simulink model "directVectorControl"  (R2021a)
settings: Solver=FixedStepAuto  StartTime=0.0  StopTime=10  FixedStep=1e-6  RelTol=1e-3
InitFcn:
  | Rs=1.405;
  | Lls=0.005839;
  | rr=1.395;
  | Llr=0.005839;
  | Lm=0.1722;
  | Lr=Llr+Lm;
  | J=0.0131;
  | B=0.002985;
  | p=4;
  | Tl=2;
  | Lr=Llr+Lm;
  | Taur=Lr/rr;
  | P = p;
  | Ls = Lls + Lm;
  | Lr = Llr + Lm;
  | Rr = rr;
  | w_frame = 2*pi*50;
  | Vdc=650;
  | car_freq=10000;
  | Rotor_Flux=0.9;
  | Delta=0.1;
libraries: pid_lib x14, spsIGBTDiodeLib x6, spsabctodq0Lib x5, eeStairGenerator x3, spsdq0toabcLib x3, spsVoltageMeasurementLib x3, spsGroundLib x2, spsDCVoltageSourceLib x1, spsAsynchronousMachineSIUnitsLib x1, spsTriangleGeneratorLib x1, spspowerguiLib x1
(part 2 of 2)

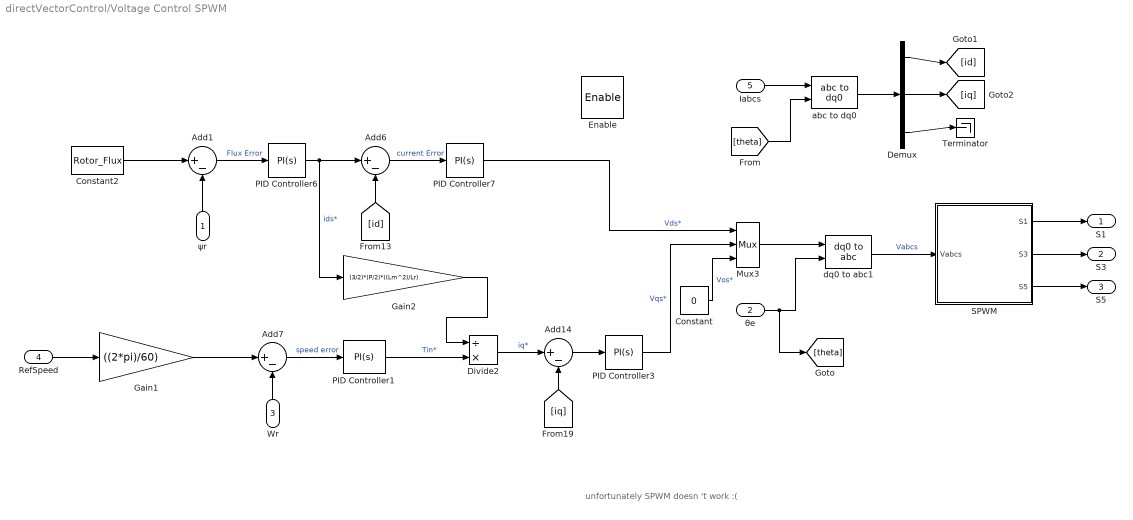
== system directVectorControl/Voltage Control SPWM ==
  note: unfortunately SPWM doesn 't work :(
  ψr : Inport
  θe : Inport  Port=2
  Wr : Inport  Port=3
  RefSpeed : Inport  Port=4
  Iabcs : Inport  Port=5
  Enable : EnablePort
  Add{1,6..7,14} (4 alike) : Sum  Inputs=|+-
  Constant : Constant  Value=0
  Constant2 : Constant  Value=Rotor_Flux
  Demux : Demux  Outputs=3
  Divide2 : Product  Inputs=/*
  Gain1 : Gain  Gain=((2*pi)/60)
  Gain2 : Gain  Gain=(3/2)*(P/2)*((Lm^2)/Lr)
  Mux3 : Mux  Inputs=3
      settings: DisplayOption=signals
  PID Controller1 : pid_lib/PID Controller  Controller=PI  Form=Parallel  TimeDomain=Continuous-time  UseExternalTs=off  SampleTime=-1  IntegratorMethod=Forward Euler  FilterMethod=Forward Euler  ControllerParametersSource=internal  P=107.29735671651  I=38872.1307396283  D=0  UseFilter=on  N=100  TunerSelectOption=Transfer Function Based (PID Tuner App)  InitialConditionSource=internal  InitialConditionForIntegrator=0  InitialConditionForFilter=0  DifferentiatorICPrevScaledInput=0  ExternalReset=none  TrackingMode=off  Kt=1  LimitOutput=off  SatLimitsSource=internal  UpperSaturationLimit=26  LowerSaturationLimit=0  LinearizeAsGain=on  AntiWindupMode=none  Kb=1  POutMin=[]  POutMax=[]  IOutMin=[]  IOutMax=[]  DOutMin=[]  DOutMax=[]  NOutMin=[]  NOutMax=[]  SumOutMin=[]  SumOutMax=[]  SaturationOutMin=[]  SaturationOutMax=[]  PParamMin=[]  PParamMax=[]  IParamMin=[]  IParamMax=[]  DParamMin=[]  DParamMax=[]  NParamMin=[]  NParamMax=[]  KbParamMin=[]  KbParamMax=[]  KtParamMin=[]  KtParamMax=[]  KbOutMin=[]  KbOutMax=[]  KtOutMin=[]  KtOutMax=[]  IntegratorOutMin=[]  IntegratorOutMax=[]  FilterOutMin=[]  FilterOutMax=[]  SumI1OutMin=[]  SumI1OutMax=[]  SumI2OutMin=[]  SumI2OutMax=[]  SumI3OutMin=[]  SumI3OutMax=[]  SumI4OutMin=[]  SumI4OutMax=[]  SumDOutMin=[]  SumDOutMax=[]  DifferentiatorOutMin=[]  DifferentiatorOutMax=[]  FilterDiffOutCoefMin=[]  FilterDiffOutCoefMax=[]  ReciprocalOutMin=[]  ReciprocalOutMax=[]  SumDenOutMin=[]  SumDenOutMax=[]  SumNumOutMin=[]  SumNumOutMax=[]  DivideOutMin=[]  DivideOutMax=[]  UdiffTsProdOutMin=[]  UdiffTsProdOutMax=[]  NTsProdOutMin=[]  NTsProdOutMax=[]  UintegralTsProdOutMin=[]  UintegralTsProdOutMax=[]  UngainTsProdOutMin=[]  UngainTsProdOutMax=[]  IntegratorContinuousStateAttributes=''  IntegratorStateMustResolveToSignalObject=off  IntegratorRTWStateStorageClass=Auto  FilterContinuousStateAttributes=''  FilterStateMustResolveToSignalObject=off  FilterRTWStateStorageClass=Auto  ParallelPVariant=InternalParameters  IdealPVariant=Disabled  IVariant=InternalParameters  DVariant=Disabled  IntegratorVariant=Continuous  SatVariant=Disabled  AWVariant=Passthrough  PCopyVariant=Disabled  TRVariant=Disabled  FdbkBlocksVariant=Forward  IdealPFdbkVariant=Disabled  SatFdbkVariant=Disabled  DerivativeFilterVariant=Disabled  NVariant=Disabled  NCopyVariant=Disabled_SignalSpec  FilterICVariant=Disabled  IntegratorICVariant=InternalICs  ExternalResetVariant=Disabled  TRSumVariant=Passthrough  SumFdbkVariant=Disabled  SumVariant=Sum_PI  TsampFilterVariant=InternalTs  TsampNgainVariant=Passthrough  TsampIntegralVariant=Passthrough  ExternalSaturationOutDataTypeStr=Inherit: Same as second input
  PID Controller3 : pid_lib/PID Controller  Controller=PI  Form=Parallel  TimeDomain=Continuous-time  UseExternalTs=off  SampleTime=-1  IntegratorMethod=Forward Euler  FilterMethod=Forward Euler  ControllerParametersSource=internal  P=417.900587639527  I=299199.169732292  D=0  UseFilter=on  N=100  TunerSelectOption=Transfer Function Based (PID Tuner App)  InitialConditionSource=internal  InitialConditionForIntegrator=0  InitialConditionForFilter=0  DifferentiatorICPrevScaledInput=0  ExternalReset=none  TrackingMode=off  Kt=1  LimitOutput=off  SatLimitsSource=internal  UpperSaturationLimit=inf  LowerSaturationLimit=-inf  LinearizeAsGain=on  AntiWindupMode=none  Kb=1  POutMin=[]  POutMax=[]  IOutMin=[]  IOutMax=[]  DOutMin=[]  DOutMax=[]  NOutMin=[]  NOutMax=[]  SumOutMin=[]  SumOutMax=[]  SaturationOutMin=[]  SaturationOutMax=[]  PParamMin=[]  PParamMax=[]  IParamMin=[]  IParamMax=[]  DParamMin=[]  DParamMax=[]  NParamMin=[]  NParamMax=[]  KbParamMin=[]  KbParamMax=[]  KtParamMin=[]  KtParamMax=[]  KbOutMin=[]  KbOutMax=[]  KtOutMin=[]  KtOutMax=[]  IntegratorOutMin=[]  IntegratorOutMax=[]  FilterOutMin=[]  FilterOutMax=[]  SumI1OutMin=[]  SumI1OutMax=[]  SumI2OutMin=[]  SumI2OutMax=[]  SumI3OutMin=[]  SumI3OutMax=[]  SumI4OutMin=[]  SumI4OutMax=[]  SumDOutMin=[]  SumDOutMax=[]  DifferentiatorOutMin=[]  DifferentiatorOutMax=[]  FilterDiffOutCoefMin=[]  FilterDiffOutCoefMax=[]  ReciprocalOutMin=[]  ReciprocalOutMax=[]  SumDenOutMin=[]  SumDenOutMax=[]  SumNumOutMin=[]  SumNumOutMax=[]  DivideOutMin=[]  DivideOutMax=[]  UdiffTsProdOutMin=[]  UdiffTsProdOutMax=[]  NTsProdOutMin=[]  NTsProdOutMax=[]  UintegralTsProdOutMin=[]  UintegralTsProdOutMax=[]  UngainTsProdOutMin=[]  UngainTsProdOutMax=[]  IntegratorContinuousStateAttributes=''  IntegratorStateMustResolveToSignalObject=off  IntegratorRTWStateStorageClass=Auto  FilterContinuousStateAttributes=''  FilterStateMustResolveToSignalObject=off  FilterRTWStateStorageClass=Auto  ParallelPVariant=InternalParameters  IdealPVariant=Disabled  IVariant=InternalParameters  DVariant=Disabled  IntegratorVariant=Continuous  SatVariant=Disabled  AWVariant=Passthrough  PCopyVariant=Disabled  TRVariant=Disabled  FdbkBlocksVariant=Forward  IdealPFdbkVariant=Disabled  SatFdbkVariant=Disabled  DerivativeFilterVariant=Disabled  NVariant=Disabled  NCopyVariant=Disabled_SignalSpec  FilterICVariant=Disabled  IntegratorICVariant=InternalICs  ExternalResetVariant=Disabled  TRSumVariant=Passthrough  SumFdbkVariant=Disabled  SumVariant=Sum_PI  TsampFilterVariant=InternalTs  TsampNgainVariant=Passthrough  TsampIntegralVariant=Passthrough  ExternalSaturationOutDataTypeStr=Inherit: Same as second input
  PID Controller6 : pid_lib/PID Controller  Controller=PI  Form=Parallel  TimeDomain=Continuous-time  UseExternalTs=off  SampleTime=-1  IntegratorMethod=Forward Euler  FilterMethod=Forward Euler  ControllerParametersSource=internal  P=1630.03954669268  I=566675.517481641  D=0  UseFilter=on  N=100  TunerSelectOption=Transfer Function Based (PID Tuner App)  InitialConditionSource=internal  InitialConditionForIntegrator=0  InitialConditionForFilter=0  DifferentiatorICPrevScaledInput=0  ExternalReset=none  TrackingMode=off  Kt=1  LimitOutput=off  SatLimitsSource=internal  UpperSaturationLimit=inf  LowerSaturationLimit=-inf  LinearizeAsGain=on  AntiWindupMode=none  Kb=1  POutMin=[]  POutMax=[]  IOutMin=[]  IOutMax=[]  DOutMin=[]  DOutMax=[]  NOutMin=[]  NOutMax=[]  SumOutMin=[]  SumOutMax=[]  SaturationOutMin=[]  SaturationOutMax=[]  PParamMin=[]  PParamMax=[]  IParamMin=[]  IParamMax=[]  DParamMin=[]  DParamMax=[]  NParamMin=[]  NParamMax=[]  KbParamMin=[]  KbParamMax=[]  KtParamMin=[]  KtParamMax=[]  KbOutMin=[]  KbOutMax=[]  KtOutMin=[]  KtOutMax=[]  IntegratorOutMin=[]  IntegratorOutMax=[]  FilterOutMin=[]  FilterOutMax=[]  SumI1OutMin=[]  SumI1OutMax=[]  SumI2OutMin=[]  SumI2OutMax=[]  SumI3OutMin=[]  SumI3OutMax=[]  SumI4OutMin=[]  SumI4OutMax=[]  SumDOutMin=[]  SumDOutMax=[]  DifferentiatorOutMin=[]  DifferentiatorOutMax=[]  FilterDiffOutCoefMin=[]  FilterDiffOutCoefMax=[]  ReciprocalOutMin=[]  ReciprocalOutMax=[]  SumDenOutMin=[]  SumDenOutMax=[]  SumNumOutMin=[]  SumNumOutMax=[]  DivideOutMin=[]  DivideOutMax=[]  UdiffTsProdOutMin=[]  UdiffTsProdOutMax=[]  NTsProdOutMin=[]  NTsProdOutMax=[]  UintegralTsProdOutMin=[]  UintegralTsProdOutMax=[]  UngainTsProdOutMin=[]  UngainTsProdOutMax=[]  IntegratorContinuousStateAttributes=''  IntegratorStateMustResolveToSignalObject=off  IntegratorRTWStateStorageClass=Auto  FilterContinuousStateAttributes=''  FilterStateMustResolveToSignalObject=off  FilterRTWStateStorageClass=Auto  ParallelPVariant=InternalParameters  IdealPVariant=Disabled  IVariant=InternalParameters  DVariant=Disabled  IntegratorVariant=Continuous  SatVariant=Disabled  AWVariant=Passthrough  PCopyVariant=Disabled  TRVariant=Disabled  FdbkBlocksVariant=Forward  IdealPFdbkVariant=Disabled  SatFdbkVariant=Disabled  DerivativeFilterVariant=Disabled  NVariant=Disabled  NCopyVariant=Disabled_SignalSpec  FilterICVariant=Disabled  IntegratorICVariant=InternalICs  ExternalResetVariant=Disabled  TRSumVariant=Passthrough  SumFdbkVariant=Disabled  SumVariant=Sum_PI  TsampFilterVariant=InternalTs  TsampNgainVariant=Passthrough  TsampIntegralVariant=Passthrough  ExternalSaturationOutDataTypeStr=Inherit: Same as second input
  PID Controller7 : pid_lib/PID Controller  Controller=PI  Form=Parallel  TimeDomain=Continuous-time  UseExternalTs=off  SampleTime=-1  IntegratorMethod=Forward Euler  FilterMethod=Forward Euler  ControllerParametersSource=internal  P=15.9312047333312  I=78964.3934467361  D=0  UseFilter=on  N=100  TunerSelectOption=Transfer Function Based (PID Tuner App)  InitialConditionSource=internal  InitialConditionForIntegrator=0  InitialConditionForFilter=0  DifferentiatorICPrevScaledInput=0  ExternalReset=none  TrackingMode=off  Kt=1  LimitOutput=off  SatLimitsSource=internal  UpperSaturationLimit=inf  LowerSaturationLimit=-inf  LinearizeAsGain=on  AntiWindupMode=none  Kb=1  POutMin=[]  POutMax=[]  IOutMin=[]  IOutMax=[]  DOutMin=[]  DOutMax=[]  NOutMin=[]  NOutMax=[]  SumOutMin=[]  SumOutMax=[]  SaturationOutMin=[]  SaturationOutMax=[]  PParamMin=[]  PParamMax=[]  IParamMin=[]  IParamMax=[]  DParamMin=[]  DParamMax=[]  NParamMin=[]  NParamMax=[]  KbParamMin=[]  KbParamMax=[]  KtParamMin=[]  KtParamMax=[]  KbOutMin=[]  KbOutMax=[]  KtOutMin=[]  KtOutMax=[]  IntegratorOutMin=[]  IntegratorOutMax=[]  FilterOutMin=[]  FilterOutMax=[]  SumI1OutMin=[]  SumI1OutMax=[]  SumI2OutMin=[]  SumI2OutMax=[]  SumI3OutMin=[]  SumI3OutMax=[]  SumI4OutMin=[]  SumI4OutMax=[]  SumDOutMin=[]  SumDOutMax=[]  DifferentiatorOutMin=[]  DifferentiatorOutMax=[]  FilterDiffOutCoefMin=[]  FilterDiffOutCoefMax=[]  ReciprocalOutMin=[]  ReciprocalOutMax=[]  SumDenOutMin=[]  SumDenOutMax=[]  SumNumOutMin=[]  SumNumOutMax=[]  DivideOutMin=[]  DivideOutMax=[]  UdiffTsProdOutMin=[]  UdiffTsProdOutMax=[]  NTsProdOutMin=[]  NTsProdOutMax=[]  UintegralTsProdOutMin=[]  UintegralTsProdOutMax=[]  UngainTsProdOutMin=[]  UngainTsProdOutMax=[]  IntegratorContinuousStateAttributes=''  IntegratorStateMustResolveToSignalObject=off  IntegratorRTWStateStorageClass=Auto  FilterContinuousStateAttributes=''  FilterStateMustResolveToSignalObject=off  FilterRTWStateStorageClass=Auto  ParallelPVariant=InternalParameters  IdealPVariant=Disabled  IVariant=InternalParameters  DVariant=Disabled  IntegratorVariant=Continuous  SatVariant=Disabled  AWVariant=Passthrough  PCopyVariant=Disabled  TRVariant=Disabled  FdbkBlocksVariant=Forward  IdealPFdbkVariant=Disabled  SatFdbkVariant=Disabled  DerivativeFilterVariant=Disabled  NVariant=Disabled  NCopyVariant=Disabled_SignalSpec  FilterICVariant=Disabled  IntegratorICVariant=InternalICs  ExternalResetVariant=Disabled  TRSumVariant=Passthrough  SumFdbkVariant=Disabled  SumVariant=Sum_PI  TsampFilterVariant=InternalTs  TsampNgainVariant=Passthrough  TsampIntegralVariant=Passthrough  ExternalSaturationOutDataTypeStr=Inherit: Same as second input
  SPWM : Subsystem
  Terminator : Terminator
  abc to dq0 : spsabctodq0Lib/abc to dq0  Alignment=90 degrees behind phase A axis
  dq0 to abc1 : spsdq0toabcLib/dq0 to abc  Alignment=90 degrees behind phase A axis
  S1 : Outport
  S3 : Outport  Port=2
  S5 : Outport  Port=3
  wires:
  [iq] -> Add14/2
  SPWM/1(S1) -> S1/1
  PID Controller1/1 -> Divide2/2  "Tin*"
  SPWM/2(S3) -> S3/1
  Mux3/1 -> dq0 to abc1/1
  Constant2/1 -> Add1/1
  Add1/1 -> PID Controller6/1  "Flux Error"
  RefSpeed/1 -> Gain1/1
  PID Controller3/1 -> Mux3/2  "Vqs*"
  Add14/1 -> PID Controller3/1
  θe/1 -> [theta], dq0 to abc1/2
  dq0 to abc1/1 -> SPWM/1(Vabcs)  "Vabcs"
  SPWM/3(S5) -> S5/1
  Constant/1 -> Mux3/3  "Vos*"
  [id] -> Add6/2
  Gain2/1 -> Divide2/1
  Gain1/1 -> Add7/1
  Add6/1 -> PID Controller7/1  "current Error"
  PID Controller7/1 -> Mux3/1  "Vds*"
  PID Controller6/1 -> Add6/1, Gain2/1  "ids*"
  Wr/1 -> Add7/2
  Divide2/1 -> Add14/1  "iq*"
  ψr/1 -> Add1/2
  Add7/1 -> PID Controller1/1  "speed error"
  Iabcs/1 -> abc to dq0/1
  [theta] -> abc to dq0/2
  abc to dq0/1 -> Demux/1
  Demux/1 -> [id]
  Demux/2 -> [iq]
  Demux/3 -> Terminator/1

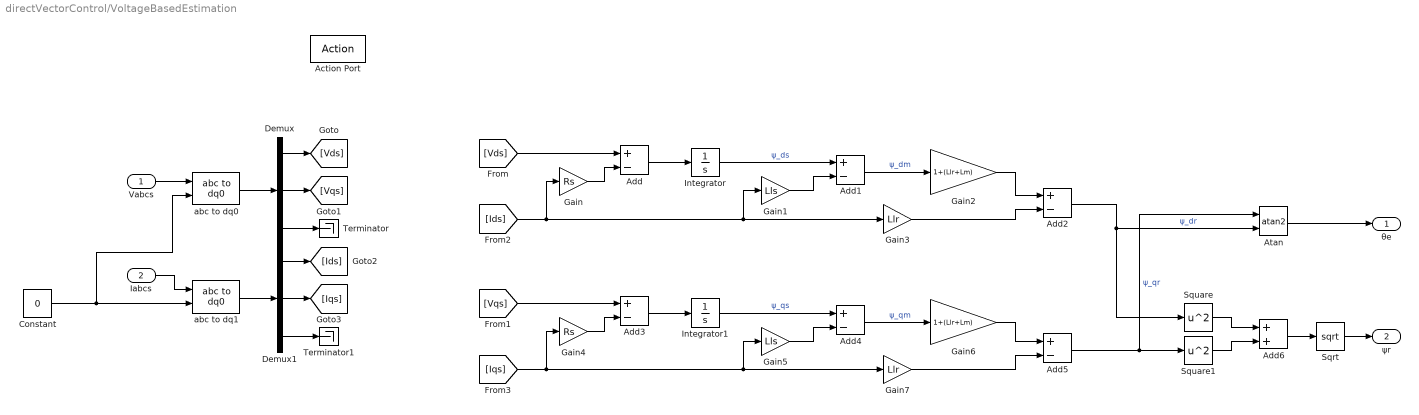
== system directVectorControl/VoltageBasedEstimation ==
  Vabcs : Inport
  Iabcs : Inport  Port=2
  Action Port : ActionPort  ActionPortLabel=else
  Add{,1..5} (6 alike) : Sum  Inputs=+-
  Add6 : Sum
  Atan : Trigonometry  Operator=atan2
  Constant : Constant  Value=0
  Demux : Demux  Outputs=3
  Demux1 : Demux  Outputs=3
  Gain : Gain  Gain=Rs
  Gain1 : Gain  Gain=Lls
  Gain2 : Gain  Gain=1+(Llr+Lm)
  Gain3 : Gain  Gain=Llr
  Gain4 : Gain  Gain=Rs
  Gain5 : Gain  Gain=Lls
  Gain6 : Gain  Gain=1+(Llr+Lm)
  Gain7 : Gain  Gain=Llr
  Integrator : Integrator
  Integrator1 : Integrator
  Sqrt : Sqrt  SaturateOnIntegerOverflow=on
  Square : Math  Operator=square  SaturateOnIntegerOverflow=on
  Square1 : Math  Operator=square  SaturateOnIntegerOverflow=on
  Terminator : Terminator
  Terminator1 : Terminator
  abc to dq0 : spsabctodq0Lib/abc to dq0  Alignment=90 degrees behind phase A axis
  abc to dq1 : spsabctodq0Lib/abc to dq0  Alignment=90 degrees behind phase A axis
  θe : Outport
  ψr : Outport  Port=2
  wires:
  Vabcs/1 -> abc to dq0/1
  Iabcs/1 -> abc to dq1/1
  Constant/1 -> abc to dq0/2, abc to dq1/2
  abc to dq0/1 -> Demux/1
  Demux/1 -> [Vds]
  Demux/2 -> [Vqs]
  Demux/3 -> Terminator/1
  abc to dq1/1 -> Demux1/1
  Demux1/1 -> [Ids]
  Demux1/2 -> [Iqs]
  Demux1/3 -> Terminator1/1
  [Vds] -> Add/1
  Gain/1 -> Add/2
  [Ids] -> Gain3/1, Gain1/1, Gain/1
  Add/1 -> Integrator/1
  Integrator/1 -> Add1/1  "ψ_ds"
  Gain1/1 -> Add1/2
  Add1/1 -> Gain2/1  "ψ_dm"
  Gain2/1 -> Add2/1
  Gain3/1 -> Add2/2
  Gain7/1 -> Add5/2
  Gain6/1 -> Add5/1
  Add4/1 -> Gain6/1  "ψ_qm"
  Gain5/1 -> Add4/2
  Integrator1/1 -> Add4/1  "ψ_qs"
  Add3/1 -> Integrator1/1
  [Iqs] -> Gain4/1, Gain5/1, Gain7/1
  Gain4/1 -> Add3/2
  [Vqs] -> Add3/1
  Add2/1 -> Atan/2, Square/1  "ψ_dr"
  Add5/1 -> Atan/1, Square1/1  "ψ_qr"
  Atan/1 -> θe/1
  Square/1 -> Add6/1
  Square1/1 -> Add6/2
  Add6/1 -> Sqrt/1
  Sqrt/1 -> ψr/1

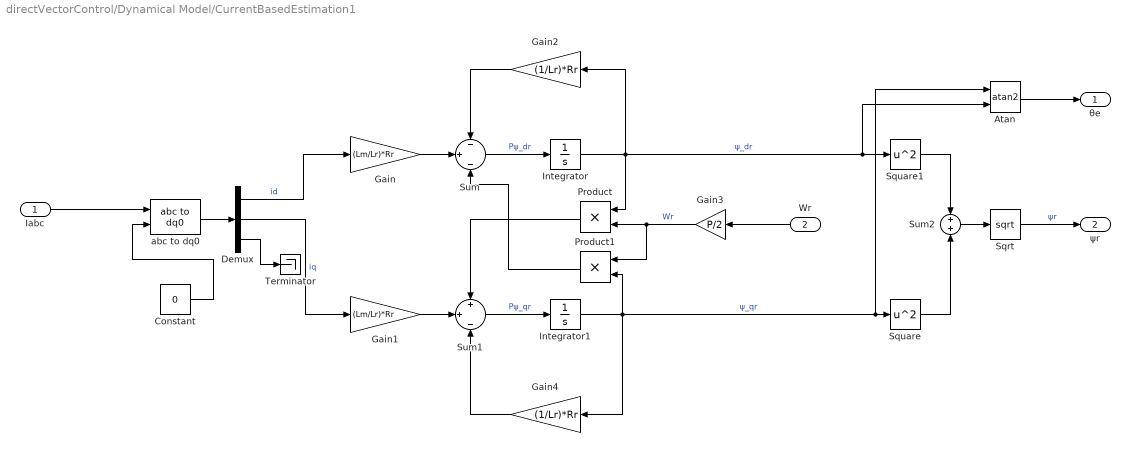
== system directVectorControl/Dynamical Model/CurrentBasedEstimation1 ==
  Iabc : Inport
  Wr : Inport  Port=2
  Atan : Trigonometry  Operator=atan2
  Constant : Constant  Value=0
  Demux : Demux  Outputs=3
  Gain : Gain  Gain=(Lm/Lr)*Rr
  Gain1 : Gain  Gain=(Lm/Lr)*Rr
  Gain2 : Gain  Gain=(1/Lr)*Rr
  Gain3 : Gain  Gain=P/2
  Gain4 : Gain  Gain=(1/Lr)*Rr
  Integrator : Integrator
  Integrator1 : Integrator
  Product : Product
  Product1 : Product
  Sqrt : Sqrt  SaturateOnIntegerOverflow=on
  Square : Math  Operator=square  SaturateOnIntegerOverflow=on
  Square1 : Math  Operator=square  SaturateOnIntegerOverflow=on
  Sum : Sum  Inputs=-|+|-
  Sum1 : Sum  Inputs=+|+|-
  Sum2 : Sum  Inputs=+|+
  Terminator : Terminator
  abc to dq0 : spsabctodq0Lib/abc to dq0  Alignment=90 degrees behind phase A axis
  θe : Outport
  ψr : Outport  Port=2
  wires:
  Integrator1/1 -> Gain4/1, Square/1, Atan/1, Product1/2  "ψ_qr"
  Integrator/1 -> Product/1, Square1/1, Atan/2, Gain2/1  "ψ_dr"
  Constant/1 -> abc to dq0/2
  Gain1/1 -> Sum1/2
  Wr/1 -> Gain3/1
  Gain2/1 -> Sum/1
  Gain/1 -> Sum/2
  Demux/1 -> Gain/1  "id"
  Gain3/1 -> Product/2, Product1/1  "Wr"
  Sum1/1 -> Integrator1/1  "Pψ_qr"
  Demux/3 -> Terminator/1
  Square/1 -> Sum2/2
  Product1/1 -> Sum/3
  abc to dq0/1 -> Demux/1
  Product/1 -> Sum1/1
  Sqrt/1 -> ψr/1  "ψr"
  Gain4/1 -> Sum1/3
  Iabc/1 -> abc to dq0/1
  Sum/1 -> Integrator/1  "Pψ_dr"
  Atan/1 -> θe/1
  Demux/2 -> Gain1/1  "iq"
  Square1/1 -> Sum2/1
  Sum2/1 -> Sqrt/1

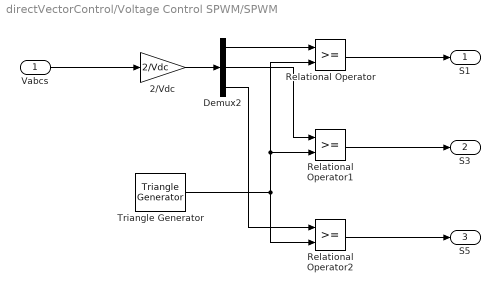
== system directVectorControl/Voltage Control SPWM/SPWM ==
  Vabcs : Inport
  2/Vdc : Gain  Gain=2/Vdc
  Demux2 : Demux  Outputs=3
  Relational Operator : RelationalOperator  OutDataTypeStr=boolean  RndMeth=Simplest
  Relational Operator1 : RelationalOperator  OutDataTypeStr=boolean  RndMeth=Simplest
  Relational Operator2 : RelationalOperator  OutDataTypeStr=boolean  RndMeth=Simplest
  Triangle Generator : spsTriangleGeneratorLib/Triangle Generator  Freq=car_freq  Phase=90  Ts=0
  S1 : Outport
  S3 : Outport  Port=2
  S5 : Outport  Port=3
  wires:
  Relational Operator1/1 -> S3/1
  Triangle Generator/1 -> Relational Operator/2, Relational Operator1/2, Relational Operator2/2
  2/Vdc/1 -> Demux2/1
  Demux2/1 -> Relational Operator/1
  Demux2/3 -> Relational Operator2/1
  Demux2/2 -> Relational Operator1/1
  Relational Operator2/1 -> S5/1
  Relational Operator/1 -> S1/1
  Vabcs/1 -> 2/Vdc/1
